simulink model "STR_lientuc"  (R2013a)
settings: Solver=ode5  SolverMode=SingleTasking  StartTime=0.0  StopTime=20  FixedStep=0.005  RelTol=1e-3
settings Model: CovMetricSettings=dwe  CovHtmlReporting=off  covSaveCumulativeToWorkspaceVar=off  CovSaveSingleToWorkspaceVar=off  CovExternalEMLEnable=on  Creator=Administrator  LastModifiedBy=Administrator
settings DataIOCC: LimitDataPoints=off  SaveFormat=StructureWithTime
settings DebuggingCC: UnderspecifiedInitializationDetection=Simplified  MergeDetectMultiDrivingBlocksExec=error  SolverPrmCheckMsg=none  FrameProcessingCompatibilityMsg=error  StateNameClashWarn=none  SFUnexpectedBacktrackingDiag=error  SFNoUnconditionalDefaultTransitionDiag=error
settings HardwareCC: ProdBitPerPointer=64  ProdLargestAtomicFloat=Float  ProdIntDivRoundTo=Zero  ProdEndianess=LittleEndian  ProdHWDeviceType=Specified
settings ModelReferenceCC: PropagateSignalLabelsOutOfModel=on
settings GRTTargetCC: CodeReplacementLibrary=C99 (ISO)  GeneratePreprocessorConditionals=Use local settings

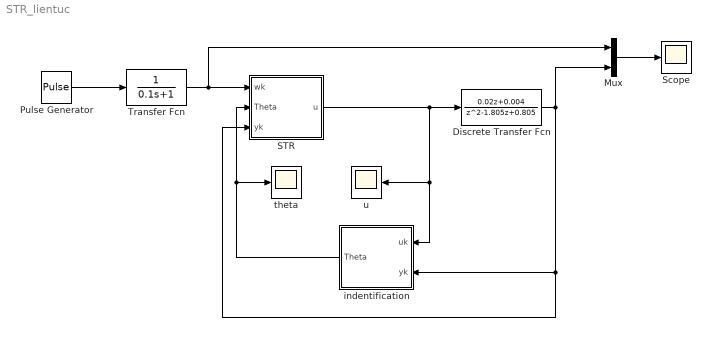
== system STR_lientuc ==
  Discrete Transfer Fcn : DiscreteTransferFcn  Numerator=[0.02 0.004]  Denominator=[1 -1.805 0.805]
  Mux : Mux  Inputs=2
  Pulse Generator : DiscretePulseGenerator  PulseType=Time based  Period=4  PulseWidth=50
  STR : Subsystem
  Scope : Scope
      settings: TimeRange=auto  MaxDataPoints=5000  SaveToWorkspace=off  SaveName=ScopeData  YMin=-0.96261  YMax=1.22067  SampleTime=-1  DataFormat=Array
  Transfer Fcn : TransferFcn  Denominator=[0.1 1]
  indentification : Subsystem
  theta : Scope
      settings: TimeRange=auto  MaxDataPoints=5000  SaveToWorkspace=off  YMin=-10  YMax=10  SampleTime=-1
  u : Scope
      settings: TimeRange=auto  LimitDataPoints=on  MaxDataPoints=5000  SaveToWorkspace=off  SaveName=ScopeData2  YMin=-10  YMax=10  SampleTime=-1  DataFormat=Array
  wires:
  Pulse Generator/1 -> Transfer Fcn/1
  Transfer Fcn/1 -> STR/1(wk), Mux/1
  STR/1(u) -> Discrete Transfer Fcn/1, indentification/1(uk), u/1
  Mux/1 -> Scope/1
  Discrete Transfer Fcn/1 -> indentification/2(yk), STR/3(yk), Mux/2
  indentification/1(Theta) -> theta/1, STR/2(Theta)

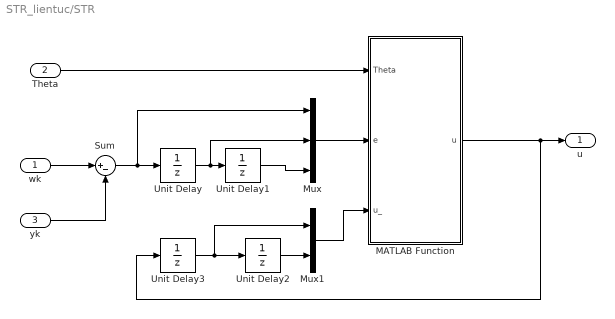
== system STR_lientuc/STR ==
  wk : Inport  PortDimensions=1
  Theta : Inport  Port=2  PortDimensions=4
  yk : Inport  Port=3  PortDimensions=1
  MATLAB Function : MATLAB Function  TreatAsAtomicUnit=on
      settings: PermitHierarchicalResolution=ParametersOnly
  Mux : Mux  Inputs=3
  Mux1 : Mux  Inputs=2
  Sum : Sum  Inputs=|+-
  Unit Delay{,1..3} (4 alike) : UnitDelay  SampleTime=-1
  u : Outport  PortDimensions=1
  wires:
  Theta/1 -> MATLAB Function/1(Theta)
  wk/1 -> Sum/1
  Sum/1 -> Mux/1, Unit Delay/1
  Unit Delay/1 -> Mux/2, Unit Delay1/1
  yk/1 -> Sum/2
  Unit Delay1/1 -> Mux/3
  Mux/1 -> MATLAB Function/2(e)
  MATLAB Function/1(u) -> Unit Delay3/1, u/1
  Unit Delay3/1 -> Mux1/1, Unit Delay2/1
  Unit Delay2/1 -> Mux1/2
  Mux1/1 -> MATLAB Function/3(u_)

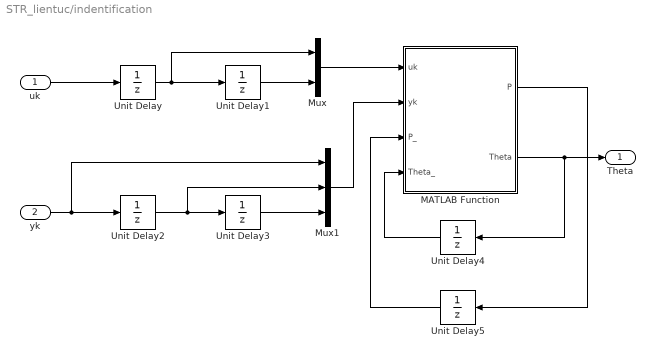
== system STR_lientuc/indentification ==
  uk : Inport  PortDimensions=1
  yk : Inport  Port=2  PortDimensions=1
  MATLAB Function : MATLAB Function  TreatAsAtomicUnit=on
      settings: PermitHierarchicalResolution=ParametersOnly
  Mux : Mux  Inputs=2
  Mux1 : Mux  Inputs=3
  Unit Delay{,1..3} (4 alike) : UnitDelay  SampleTime=-1
  Unit Delay4 : UnitDelay  InitialCondition=rand(4,1)  SampleTime=-1
  Unit Delay5 : UnitDelay  InitialCondition=1e5*eye(4)  SampleTime=-1
  Theta : Outport  PortDimensions=4
  wires:
  uk/1 -> Unit Delay/1
  Unit Delay/1 -> Mux/1, Unit Delay1/1
  Unit Delay1/1 -> Mux/2
  Mux/1 -> MATLAB Function/1(uk)
  Unit Delay3/1 -> Mux1/3
  Unit Delay2/1 -> Mux1/2, Unit Delay3/1
  yk/1 -> Mux1/1, Unit Delay2/1
  Mux1/1 -> MATLAB Function/2(yk)
  MATLAB Function/2(Theta) -> Unit Delay4/1, Theta/1
  Unit Delay4/1 -> MATLAB Function/4(Theta_)
  MATLAB Function/1(P) -> Unit Delay5/1
  Unit Delay5/1 -> MATLAB Function/3(P_)

== matlab function STR_lientuc/STR/MATLAB Function ==
  data: Theta input; u output; e input; u_ input

% Ham tinh thong so bo dieu khien theo pp dat cuc lien tuc
function u = STR_pp1(Theta,e,u_)
T0 = 0.005;
xi = 0.8;
wn = 17.5;
% Gan lai thong so de thuan tien viec tinh toan
a1 = Theta(1);
a2 = Theta(2);
b1 = Theta(3);
b2 = Theta(4);
% Tinh thong so bo dieu khien
if(xi<1)
    d1 = -2*exp(-xi*wn*T0)*cos(wn*T0*sqrt(1-xi^2)); % xi<1
else
    d1 = -2*exp(-xi*wn*T0)*cosh(wn*T0*sqrt(1-xi^2)); % xi>1
end
d2 = exp(-2*xi*wn*T0);
r1 = (b1+b2)*(a1*b1*b2-a2*(b1^2)-b2^2);
s1 = a2*((b1+b2)*(a1*b2-a2*b1)+b2*(b1*d2-b2*d1-b2));
q2 = s1/r1;
gamma = q2*(b2/a2);
q1 = (a2/b2)-q2*(b1/b2-a1/a2+1);
q0 = (1/b1)*(d1+1-a1-gamma);
% Luat dieu khien
u = q0*e(1) + q1*e(2) + q2*e(3) + (1-gamma)*u_(1) + gamma*u_(2);

== matlab function STR_lientuc/indentification/MATLAB Function ==
  data: uk input; P output; yk input; P_ input; Theta_ input; Theta output
% Ham nhan dang thong so doi tuong
function [P,Theta] = Uocluong(uk,yk,P_,Theta_)
lamda = 0.96;
PHI = [-yk(2); -yk(3); uk(1); uk(2)];
e = yk(1) - PHI'*Theta_;
L = P_*PHI / (lamda + PHI'*P_*PHI);
P = 1/lamda*(P_ - P_*PHI*PHI'*P_ /(lamda + PHI'*P_*PHI));
Theta = Theta_ + L*e;
